simulink model "Kessler"  (R2018a)
settings: Solver=VariableStepAuto  StartTime=0.0  StopTime=100  RelTol=1e-3
settings Model: Creator=benko  LastModifiedBy=benko

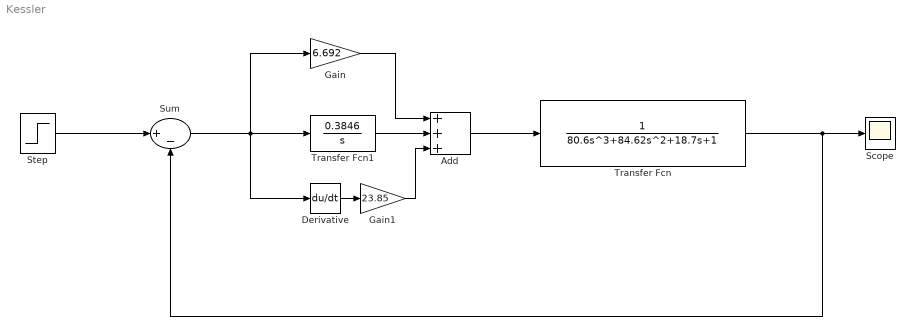
== system Kessler ==
  Add : Sum  Inputs=+++
  Derivative : Derivative
  Gain : Gain  Gain=6.692
  Gain1 : Gain  Gain=23.85
  Scope : Scope
  Step : Step  SampleTime=0
  Sum : Sum  Inputs=|+-
  Transfer Fcn : TransferFcn  Numerator=1  Denominator=[80.6 84.62 18.7 1]
  Transfer Fcn1 : TransferFcn  Numerator=[0 0.3846]  Denominator=[1 0]
  wires:
  Transfer Fcn/1 -> Sum/2, Scope/1
  Step/1 -> Sum/1
  Add/1 -> Transfer Fcn/1
  Gain/1 -> Add/1
  Transfer Fcn1/1 -> Add/2
  Derivative/1 -> Gain1/1
  Gain1/1 -> Add/3
  Sum/1 -> Gain/1, Derivative/1, Transfer Fcn1/1
